simulink model "FM"  (R2020a)
settings: Solver=VariableStepAuto  StartTime=0.0  StopTime=10.0  RelTol=1e-3
settings Model: Creator=shahb  LastModifiedBy=shahb

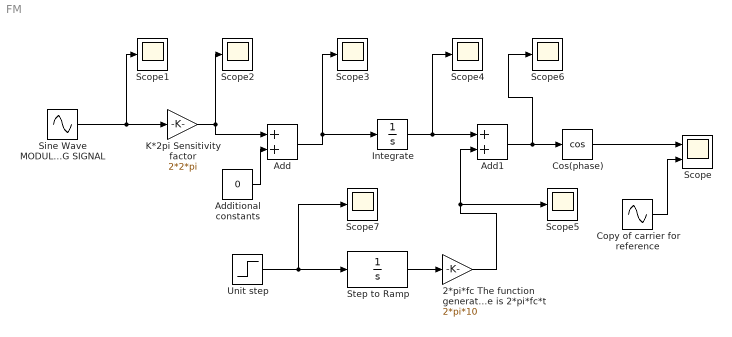
== system FM ==
  2*pi*fc The function generated till here is 2*pi*fc*t : Gain  Gain=2*pi*10
  Add : Sum
  Add1 : Sum
  Additional constants : Constant  Value=0
  Copy of carrier for reference : Sin  Frequency=2*pi*10  Phase=pi/2  SampleTime=1/5000
  Cos(phase) : Trigonometry  Operator=cos
  Integrate : Integrator
  K*2pi Sensitivity factor : Gain  Gain=2*2*pi
  Scope : Scope  NumInputPorts=2
  Scope{1..7} (7 alike) : Scope
  Sine Wave MODULATING SIGNAL : Sin  Frequency=2*pi*2  Phase=pi/2  SampleTime=1/5000
  Step to Ramp : TransferFcn  Denominator=[1 0]
  Unit step : Step  Time=0  SampleTime=1/5000
  wires:
  Sine Wave MODULATING SIGNAL/1 -> Scope1/1, K*2pi Sensitivity factor/1
  K*2pi Sensitivity factor/1 -> Scope2/1, Add/1
  Additional constants/1 -> Add/2
  Add/1 -> Scope3/1, Integrate/1
  Integrate/1 -> Add1/1, Scope4/1
  Cos(phase)/1 -> Scope/1
  Unit step/1 -> Step to Ramp/1, Scope7/1
  2*pi*fc The function generated till here is 2*pi*fc*t/1 -> Add1/2, Scope5/1
  Step to Ramp/1 -> 2*pi*fc The function generated till here is 2*pi*fc*t/1
  Add1/1 -> Scope6/1, Cos(phase)/1
  Copy of carrier for reference/1 -> Scope/2
